simulink library "PD_Controller_Lib"  (R2018b)
settings: Solver=VariableStepAuto  StartTime=0.0  StopTime=10.0  RelTol=1e-3
undefined symbols (not defined in the file): Kd, Kp
libraries: aerolibutil x2
settings Model: Creator=devantormey  LastModifiedBy=devantormey

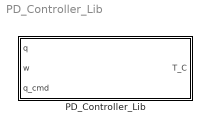
== system PD_Controller_Lib ==
  PD_Controller_Lib : Subsystem

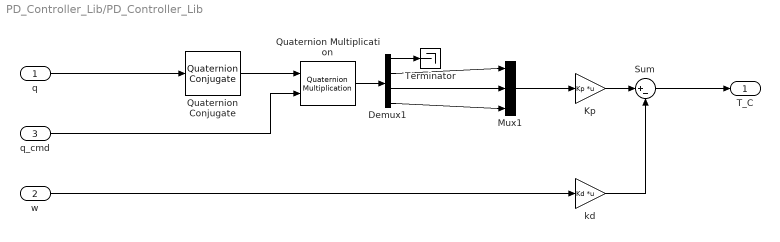
== system PD_Controller_Lib/PD_Controller_Lib ==
  q : Inport
  w : Inport  Port=2
  q_cmd : Inport  Port=3
  Demux1 : Demux
  Kp : Gain  Gain=Kp  Multiplication=Matrix(K*u)
  Mux1 : Mux  Inputs=3
  Quaternion Conjugate : aerolibutil/Quaternion Conjugate
      settings: SourceProductName=Aerospace Blockset  SourceProductBaseCode=AE
  Quaternion Multiplication : aerolibutil/Quaternion Multiplication
  Sum : Sum  Inputs=|+-
  Terminator : Terminator
  kd : Gain  Gain=Kd  Multiplication=Matrix(K*u)
  T_C : Outport
  wires:
  q/1 -> Quaternion Conjugate/1
  Demux1/3 -> Mux1/2
  Kp/1 -> Sum/1
  Demux1/4 -> Mux1/3
  w/1 -> kd/1
  Sum/1 -> T_C/1
  Mux1/1 -> Kp/1
  Demux1/2 -> Mux1/1
  q_cmd/1 -> Quaternion Multiplication/2
  Quaternion Conjugate/1 -> Quaternion Multiplication/1
  kd/1 -> Sum/2
  Quaternion Multiplication/1 -> Demux1/1
  Demux1/1 -> Terminator/1
